simulink model "e4"  (R2016b)
settings: Solver=FixedStepDiscrete  StartTime=0.0  StopTime=inf  FixedStep=0.025  RelTol=1e-3  EnableMultiTasking=on
undefined symbols (not defined in the file or in its folder): codertarget, gcbh, sigbuilder_block
libraries: arduinolib x9, simulink x8, RASPlib x3, MinSegLibrary_M1V4 x3
settings Model: SimulationMode=external  ExtModeTrigDuration=2  Creator=Hamza  LastModifiedBy=Hamza
settings OptimizationCC: MaxStackSize=64
settings DebuggingCC: ParameterTunabilityLossMsg=error
settings HardwareCC: ProdBitPerPointer=32  ProdBitPerSizeT=32  ProdBitPerPtrDiffT=32  ProdLargestAtomicInteger=Long  ProdLargestAtomicFloat=Double  ProdWordSize=32  ProdHWDeviceType=ARM Compatible->ARM Cortex
settings RTWCC: SystemTargetFile=ert.tlc  HardwareBoard=Arduino Due  TLCOptions=-aInlineSetEventsForThisBaseRateFcn=TLC_FALSE -aSuppressMultiTaskScheduler=TLC_FALSE -aRateBasedStepFcn=1  TemplateMakefile=ert_default_tmf  Description=Embedded Coder  GenerateReport=on  Toolchain=Arduino ARM  BuildConfiguration=Faster Runs  IncludeHyperlinkInReport=on  LaunchReport=on  GenerateTraceInfo=on  GenerateTraceReport=on  GenerateTraceReportSl=on  GenerateTraceReportSf=on  GenerateTraceReportEml=on
settings CodeAppCC: ForceParamTrailComments=on  IgnoreCustomStorageClasses=off  OperatorAnnotations=on  SimulinkDataObjDesc=on  SFDataObjDesc=on  MATLABFcnDesc=on  InsertBlockDesc=on  MATLABSourceComments=on
settings ERTTargetCC: SupportContinuousTime=on  SupportVariableSizeSignals=on

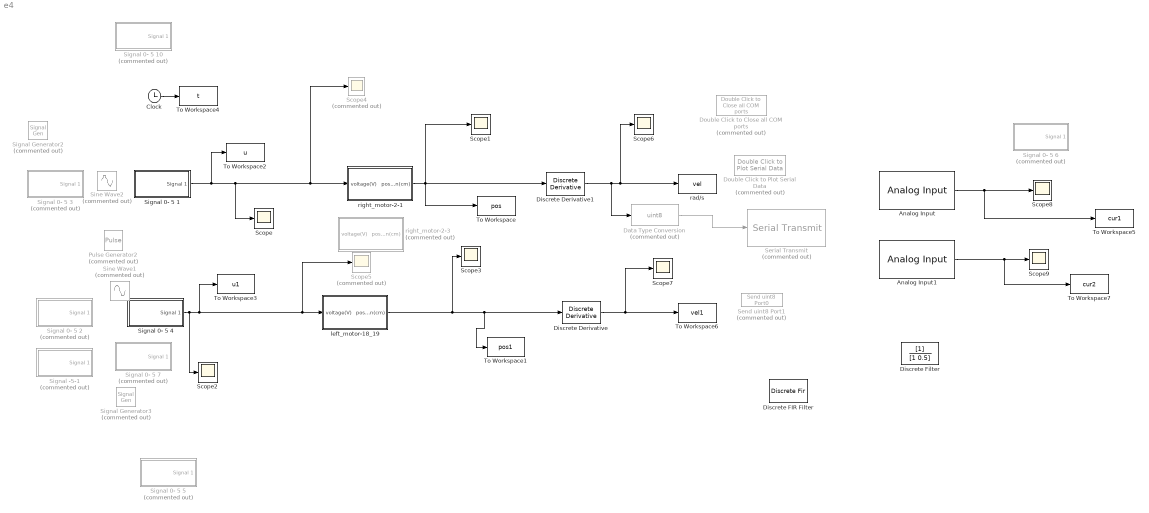
== system e4 ==
  Analog Input : arduinolib/Analog Input  pinNumber=0  sampleTime=0.025  blockPlatform=arduino
  Analog Input1 : arduinolib/Analog Input  pinNumber=1  sampleTime=0.025  blockPlatform=arduino
  Clock : Clock
  Data Type Conversion : DataTypeConversion  Commented=on  OutDataTypeStr=uint8
  Discrete Derivative : simulink/Discrete/Discrete Derivative  gainval=1.0  ICPrevScaledInput=0.0  OutMin=[]  OutMax=[]  OutDataType=fixdt(1, 16)  OutScaling=2^-10  DoSatur=off
  Discrete Derivative1 : simulink/Discrete/Discrete Derivative  gainval=1.0  ICPrevScaledInput=0.0  OutMin=[]  OutMax=[]  OutDataType=fixdt(1, 16)  OutScaling=2^-10  DoSatur=off
  Discrete FIR Filter : DiscreteFir
  Discrete Filter : DiscreteFilter
  Double Click to Close all COM ports : RASPlib/Double Click to Close all COM ports  Commented=on
  Double Click to Plot Serial Data : RASPlib/Double Click to Plot Serial Data  Commented=on  COMport=3  BaudRate=115200  NumSamples=10000  DataType=uint8
  Pulse Generator2 : DiscretePulseGenerator  Commented=on  PulseType=Time based  Amplitude=5  Period=20  PulseWidth=50  PhaseDelay=5
  Scope{,1..3,6..9} (8 alike) : Scope
  Scope4 : Scope  Commented=on
  Scope5 : Scope  Commented=on
  Send uint8 Port1 : RASPlib/Send uint8 Port0  Commented=on
  Serial Transmit : arduinolib/Serial Transmit  Commented=on  portNumber=0  blockPlatform=arduino
  Signal Generator2 : SignalGenerator  Commented=on  WaveForm=sawtooth  Amplitude=5  Frequency=0.05*pi  Units=rad/sec
  Signal Generator3 : SignalGenerator  Commented=on  WaveForm=sawtooth  Amplitude=-5  Frequency=0.05*pi  Units=rad/sec
  Signal -5-1 : Subsystem  Tag=STV Subsys  Commented=on  LoadFcn=sigbuilder_block('load');  StartFcn=sigbuilder_block('start');  StopFcn=sigbuilder_block('stop');  ClipboardFcn=sigbuilder_block('clipboard');  mask(Sigbuilder block){tuvar=[0:10]}
      mask help: Simulink:masks:SigbuilderBlock_MD
      mask init:
      | if ~strcmp(get_param(bdroot(gcbh),'SimulationStatus'),'stopped') tuvar = sigbuilder_block('maskInit'); end
      settings: CopyFcn=sigbuilder_block('copy');  DeleteFcn=sigbuilder_block('delete');  ModelCloseFcn=sigbuilder_block('modelClose');  PreSaveFcn=sigbuilder_block('preSave');  PauseFcn=sigbuilder_block('pause');  ContinueFcn=sigbuilder_block('continue');  NameChangeFcn=sigbuilder_block('namechange');  OpenFcn=sigbuilder_block('open',[6 30 1012.5 447.75 ]);  CloseFcn=sigbuilder_block('close');
      mask Display: plot(0, 0, 100, 100,[2, 2, 32, 32, 2], [68, 8, 8, 68, 68],[32, 2], [38, 38], [32, 19, 2],[53, 60, 44], [32, 17, 17, 2],[16, 16, 31, 31]);txt = getActiveGroup(gcbh);text(2, 100, txt,'verticalAlignment', 'top');
  Signal 0- 5 1 : Subsystem  Tag=STV Subsys  LoadFcn=sigbuilder_block('load');  StartFcn=sigbuilder_block('start');  StopFcn=sigbuilder_block('stop');  ClipboardFcn=sigbuilder_block('clipboard');  mask(Sigbuilder block){tuvar=[0:10]}
      mask help: Simulink:masks:SigbuilderBlock_MD
      mask init:
      | if ~strcmp(get_param(bdroot(gcbh),'SimulationStatus'),'stopped') tuvar = sigbuilder_block('maskInit'); end
      settings: CopyFcn=sigbuilder_block('copy');  DeleteFcn=sigbuilder_block('delete');  ModelCloseFcn=sigbuilder_block('modelClose');  PreSaveFcn=sigbuilder_block('preSave');  PauseFcn=sigbuilder_block('pause');  ContinueFcn=sigbuilder_block('continue');  NameChangeFcn=sigbuilder_block('namechange');  OpenFcn=sigbuilder_block('open',[6 30 1012.5 447.75 ]);  CloseFcn=sigbuilder_block('close');
      mask Display: plot(0, 0, 100, 100,[2, 2, 32, 32, 2], [68, 8, 8, 68, 68],[32, 2], [38, 38], [32, 19, 2],[53, 60, 44], [32, 17, 17, 2],[16, 16, 31, 31]);txt = getActiveGroup(gcbh);text(2, 100, txt,'verticalAlignment', 'top');
  Signal 0- 5 10 : Subsystem  Tag=STV Subsys  Commented=on  LoadFcn=sigbuilder_block('load');  StartFcn=sigbuilder_block('start');  StopFcn=sigbuilder_block('stop');  ClipboardFcn=sigbuilder_block('clipboard');  mask(Sigbuilder block){tuvar=[0:10]}
      mask help: Simulink:masks:SigbuilderBlock_MD
      mask init:
      | if ~strcmp(get_param(bdroot(gcbh),'SimulationStatus'),'stopped') tuvar = sigbuilder_block('maskInit'); end
      settings: CopyFcn=sigbuilder_block('copy');  DeleteFcn=sigbuilder_block('delete');  ModelCloseFcn=sigbuilder_block('modelClose');  PreSaveFcn=sigbuilder_block('preSave');  PauseFcn=sigbuilder_block('pause');  ContinueFcn=sigbuilder_block('continue');  NameChangeFcn=sigbuilder_block('namechange');  OpenFcn=sigbuilder_block('open',[6 30 1012.5 447.75 ]);  CloseFcn=sigbuilder_block('close');
      mask Display: plot(0, 0, 100, 100,[2, 2, 32, 32, 2], [68, 8, 8, 68, 68],[32, 2], [38, 38], [32, 19, 2],[53, 60, 44], [32, 17, 17, 2],[16, 16, 31, 31]);txt = getActiveGroup(gcbh);text(2, 100, txt,'verticalAlignment', 'top');
  Signal 0- 5 2 : Subsystem  Tag=STV Subsys  Commented=on  LoadFcn=sigbuilder_block('load');  StartFcn=sigbuilder_block('start');  StopFcn=sigbuilder_block('stop');  ClipboardFcn=sigbuilder_block('clipboard');  mask(Sigbuilder block){tuvar=[0:10]}
      mask help: Simulink:masks:SigbuilderBlock_MD
      mask init:
      | if ~strcmp(get_param(bdroot(gcbh),'SimulationStatus'),'stopped') tuvar = sigbuilder_block('maskInit'); end
      settings: CopyFcn=sigbuilder_block('copy');  DeleteFcn=sigbuilder_block('delete');  ModelCloseFcn=sigbuilder_block('modelClose');  PreSaveFcn=sigbuilder_block('preSave');  PauseFcn=sigbuilder_block('pause');  ContinueFcn=sigbuilder_block('continue');  NameChangeFcn=sigbuilder_block('namechange');  OpenFcn=sigbuilder_block('open',[6 30 1012.5 447.75 ]);  CloseFcn=sigbuilder_block('close');
      mask Display: plot(0, 0, 100, 100,[2, 2, 32, 32, 2], [68, 8, 8, 68, 68],[32, 2], [38, 38], [32, 19, 2],[53, 60, 44], [32, 17, 17, 2],[16, 16, 31, 31]);txt = getActiveGroup(gcbh);text(2, 100, txt,'verticalAlignment', 'top');
  Signal 0- 5 3 : Subsystem  Tag=STV Subsys  Commented=on  LoadFcn=sigbuilder_block('load');  StartFcn=sigbuilder_block('start');  StopFcn=sigbuilder_block('stop');  ClipboardFcn=sigbuilder_block('clipboard');  mask(Sigbuilder block){tuvar=[0:10]}
      mask help: Simulink:masks:SigbuilderBlock_MD
      mask init:
      | if ~strcmp(get_param(bdroot(gcbh),'SimulationStatus'),'stopped') tuvar = sigbuilder_block('maskInit'); end
      settings: CopyFcn=sigbuilder_block('copy');  DeleteFcn=sigbuilder_block('delete');  ModelCloseFcn=sigbuilder_block('modelClose');  PreSaveFcn=sigbuilder_block('preSave');  PauseFcn=sigbuilder_block('pause');  ContinueFcn=sigbuilder_block('continue');  NameChangeFcn=sigbuilder_block('namechange');  OpenFcn=sigbuilder_block('open',[6 30 1012.5 447.75 ]);  CloseFcn=sigbuilder_block('close');
      mask Display: plot(0, 0, 100, 100,[2, 2, 32, 32, 2], [68, 8, 8, 68, 68],[32, 2], [38, 38], [32, 19, 2],[53, 60, 44], [32, 17, 17, 2],[16, 16, 31, 31]);txt = getActiveGroup(gcbh);text(2, 100, txt,'verticalAlignment', 'top');
  Signal 0- 5 4 : Subsystem  Tag=STV Subsys  LoadFcn=sigbuilder_block('load');  StartFcn=sigbuilder_block('start');  StopFcn=sigbuilder_block('stop');  ClipboardFcn=sigbuilder_block('clipboard');  mask(Sigbuilder block){tuvar=[0:10]}
      mask help: Simulink:masks:SigbuilderBlock_MD
      mask init:
      | if ~strcmp(get_param(bdroot(gcbh),'SimulationStatus'),'stopped') tuvar = sigbuilder_block('maskInit'); end
      settings: CopyFcn=sigbuilder_block('copy');  DeleteFcn=sigbuilder_block('delete');  ModelCloseFcn=sigbuilder_block('modelClose');  PreSaveFcn=sigbuilder_block('preSave');  PauseFcn=sigbuilder_block('pause');  ContinueFcn=sigbuilder_block('continue');  NameChangeFcn=sigbuilder_block('namechange');  OpenFcn=sigbuilder_block('open',[6 30 1012.5 447.75 ]);  CloseFcn=sigbuilder_block('close');
      mask Display: plot(0, 0, 100, 100,[2, 2, 32, 32, 2], [68, 8, 8, 68, 68],[32, 2], [38, 38], [32, 19, 2],[53, 60, 44], [32, 17, 17, 2],[16, 16, 31, 31]);txt = getActiveGroup(gcbh);text(2, 100, txt,'verticalAlignment', 'top');
  Signal 0- 5 5 : Subsystem  Tag=STV Subsys  Commented=on  LoadFcn=sigbuilder_block('load');  StartFcn=sigbuilder_block('start');  StopFcn=sigbuilder_block('stop');  ClipboardFcn=sigbuilder_block('clipboard');  mask(Sigbuilder block){tuvar=[0:10]}
      mask help: Simulink:masks:SigbuilderBlock_MD
      mask init:
      | if ~strcmp(get_param(bdroot(gcbh),'SimulationStatus'),'stopped') tuvar = sigbuilder_block('maskInit'); end
      settings: CopyFcn=sigbuilder_block('copy');  DeleteFcn=sigbuilder_block('delete');  ModelCloseFcn=sigbuilder_block('modelClose');  PreSaveFcn=sigbuilder_block('preSave');  PauseFcn=sigbuilder_block('pause');  ContinueFcn=sigbuilder_block('continue');  NameChangeFcn=sigbuilder_block('namechange');  OpenFcn=sigbuilder_block('open',[6 30 1012.5 447.75 ]);  CloseFcn=sigbuilder_block('close');
      mask Display: plot(0, 0, 100, 100,[2, 2, 32, 32, 2], [68, 8, 8, 68, 68],[32, 2], [38, 38], [32, 19, 2],[53, 60, 44], [32, 17, 17, 2],[16, 16, 31, 31]);txt = getActiveGroup(gcbh);text(2, 100, txt,'verticalAlignment', 'top');
  Signal 0- 5 6 : Subsystem  Tag=STV Subsys  Commented=on  LoadFcn=sigbuilder_block('load');  StartFcn=sigbuilder_block('start');  StopFcn=sigbuilder_block('stop');  ClipboardFcn=sigbuilder_block('clipboard');  mask(Sigbuilder block){tuvar=[0:10]}
      mask help: Simulink:masks:SigbuilderBlock_MD
      mask init:
      | if ~strcmp(get_param(bdroot(gcbh),'SimulationStatus'),'stopped') tuvar = sigbuilder_block('maskInit'); end
      settings: CopyFcn=sigbuilder_block('copy');  DeleteFcn=sigbuilder_block('delete');  ModelCloseFcn=sigbuilder_block('modelClose');  PreSaveFcn=sigbuilder_block('preSave');  PauseFcn=sigbuilder_block('pause');  ContinueFcn=sigbuilder_block('continue');  NameChangeFcn=sigbuilder_block('namechange');  OpenFcn=sigbuilder_block('open',[6 30 1012.5 447.75 ]);  CloseFcn=sigbuilder_block('close');
      mask Display: plot(0, 0, 100, 100,[2, 2, 32, 32, 2], [68, 8, 8, 68, 68],[32, 2], [38, 38], [32, 19, 2],[53, 60, 44], [32, 17, 17, 2],[16, 16, 31, 31]);txt = getActiveGroup(gcbh);text(2, 100, txt,'verticalAlignment', 'top');
  Signal 0- 5 7 : Subsystem  Tag=STV Subsys  Commented=on  LoadFcn=sigbuilder_block('load');  StartFcn=sigbuilder_block('start');  StopFcn=sigbuilder_block('stop');  ClipboardFcn=sigbuilder_block('clipboard');  mask(Sigbuilder block){tuvar=[0:10]}
      mask help: Simulink:masks:SigbuilderBlock_MD
      mask init:
      | if ~strcmp(get_param(bdroot(gcbh),'SimulationStatus'),'stopped') tuvar = sigbuilder_block('maskInit'); end
      settings: CopyFcn=sigbuilder_block('copy');  DeleteFcn=sigbuilder_block('delete');  ModelCloseFcn=sigbuilder_block('modelClose');  PreSaveFcn=sigbuilder_block('preSave');  PauseFcn=sigbuilder_block('pause');  ContinueFcn=sigbuilder_block('continue');  NameChangeFcn=sigbuilder_block('namechange');  OpenFcn=sigbuilder_block('open',[6 30 1012.5 447.75 ]);  CloseFcn=sigbuilder_block('close');
      mask Display: plot(0, 0, 100, 100,[2, 2, 32, 32, 2], [68, 8, 8, 68, 68],[32, 2], [38, 38], [32, 19, 2],[53, 60, 44], [32, 17, 17, 2],[16, 16, 31, 31]);txt = getActiveGroup(gcbh);text(2, 100, txt,'verticalAlignment', 'top');
  Sine Wave1 : Sin  Commented=on  Amplitude=5  Frequency=0.4*3.14  Phase=pi
  Sine Wave2 : Sin  Commented=on  Amplitude=5  Frequency=0.4*pi
  To Workspace : ToWorkspace  VariableName=pos  SampleTime=-1
      settings: Save2DSignal=2-D array (concatenate along first dimension)
  To Workspace1 : ToWorkspace  VariableName=pos1  SampleTime=-1
      settings: Save2DSignal=2-D array (concatenate along first dimension)
  To Workspace2 : ToWorkspace  VariableName=u  SampleTime=-1
      settings: Save2DSignal=2-D array (concatenate along first dimension)
  To Workspace3 : ToWorkspace  VariableName=u1  SampleTime=-1
      settings: Save2DSignal=2-D array (concatenate along first dimension)
  To Workspace4 : ToWorkspace  VariableName=t  SampleTime=-1
      settings: Save2DSignal=2-D array (concatenate along first dimension)
  To Workspace5 : ToWorkspace  VariableName=cur1  SampleTime=-1
      settings: Save2DSignal=2-D array (concatenate along first dimension)
  To Workspace6 : ToWorkspace  VariableName=vel1  SampleTime=-1
      settings: Save2DSignal=2-D array (concatenate along first dimension)
  To Workspace7 : ToWorkspace  VariableName=cur2  SampleTime=-1
      settings: Save2DSignal=2-D array (concatenate along first dimension)
  "left_motor-18_19 " : Subsystem
  rad/s : ToWorkspace  VariableName=vel  SampleTime=-1
      settings: Save2DSignal=2-D array (concatenate along first dimension)
  right_motor-2-1 : Subsystem
  right_motor-2-3 : Subsystem  Commented=on
  wires:
  right_motor-2-1/1(position(cm)) -> To Workspace/1, Scope1/1, Discrete Derivative1/1
  "left_motor-18_19 "/1(position(cm)) -> Discrete Derivative/1, To Workspace1/1, Scope3/1
  Signal 0- 5 4/1(Signal 1) -> Scope2/1, Scope5/1, "left_motor-18_19 "/1(voltage(V)), To Workspace3/1
  Clock/1 -> To Workspace4/1
  Discrete Derivative/1 -> Scope7/1, To Workspace6/1
  Discrete Derivative1/1 -> Data Type Conversion/1, Scope6/1, rad/s/1
  Data Type Conversion/1 -> Serial Transmit/1
  Signal 0- 5 1/1(Signal 1) -> To Workspace2/1, Scope/1, right_motor-2-1/1(voltage(V)), Scope4/1
  Analog Input/1 -> To Workspace5/1, Scope8/1
  Analog Input1/1 -> To Workspace7/1, Scope9/1

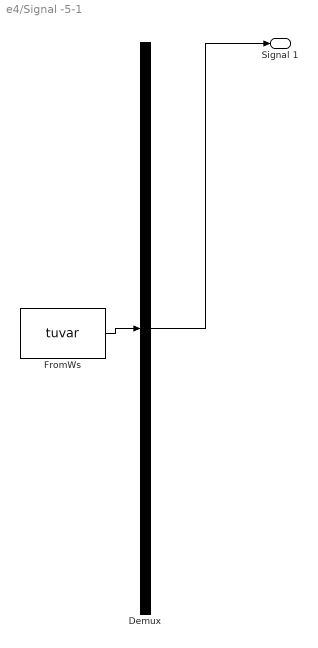
== system e4/Signal -5-1 ==
  Demux : Demux  Tag=STV Demux  Outputs=1
  FromWs : FromWorkspace  Tag=STV FromWs  VariableName=tuvar  SampleTime=0
      SigBuilderData=|
      | common.afterFinalStr = 'Extrapolate'
      | common.sampleTime = 0
      | dataSet.timeRange = [0 60]
      | dataSet.name = 'Group 1'
      | sbobj.Groups.Name = 'Group 1'
      | sbobj.Groups.Signals.Name = 'Signal 1'
      | sbobj.Groups.Signals.XData = [0 5 5 9.99 9.99 15 15 20.005 20.005 25 25 30 30 34.95 34.95 40 40 45 45 50 50 55 55 60]
      | sbobj.Groups.Signals.YData = [0 0 -5 -5 -4.5 -4.5 -4 -4 -3.49 -3.49 -3.01 -3.01 -2.49 -2.49 -2 -2 -1.5 -1.5 -1.01 -1.01 -0.5 -0.5 0 0]
      | sbobj.Groups.TimeRange = [0 60]
  Signal 1 : Outport  Tag=STV Outport
  wires:
  FromWs/1 -> Demux/1
  Demux/1 -> Signal 1/1

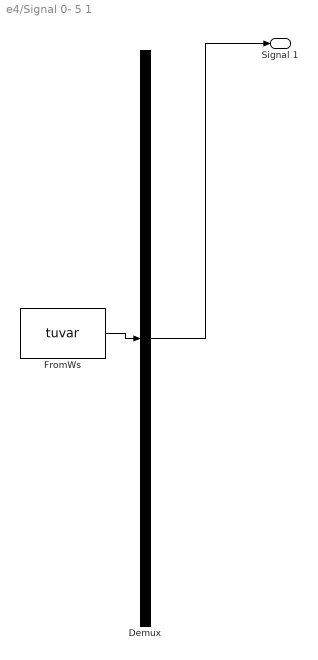
== system e4/Signal 0- 5 1 ==
  Demux : Demux  Tag=STV Demux  Outputs=1
  FromWs : FromWorkspace  Tag=STV FromWs  VariableName=tuvar  SampleTime=0
      SigBuilderData=|
      | common.afterFinalStr = 'Extrapolate'
      | common.sampleTime = 0
      | dataSet.timeRange = [0 150]
      | dataSet.name = 'Group 1'
      | sbobj.Groups.Name = 'Group 1'
      | sbobj.Groups.Signals.Name = 'Signal 1'
      | sbobj.Groups.Signals.XData = [0 5 10 15 20 25 30 35 40 45 47.5 50 52.5 55 57.5 60 62.5 70 75 80 85 90 95 100 105 150]
      | sbobj.Groups.Signals.YData = [0 0 5 5 0 0 -5 -5 0 0 5 5 0 0 -5 -5 0 0 -5 -5 0 0 5 5 0 0]
      | sbobj.Groups.TimeRange = [0 150]
  Signal 1 : Outport  Tag=STV Outport
  wires:
  FromWs/1 -> Demux/1
  Demux/1 -> Signal 1/1

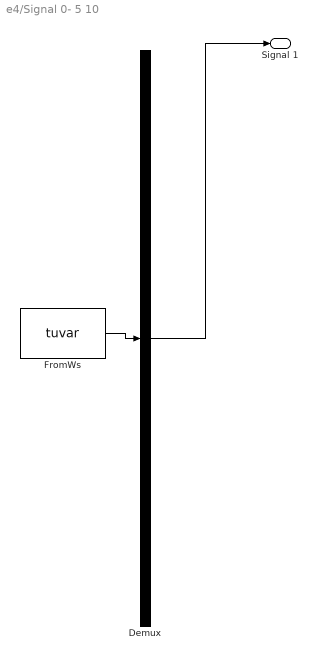
== system e4/Signal 0- 5 10 ==
  Demux : Demux  Tag=STV Demux  Outputs=1
  FromWs : FromWorkspace  Tag=STV FromWs  VariableName=tuvar  SampleTime=0
      SigBuilderData=|
      | common.afterFinalStr = 'Extrapolate'
      | common.sampleTime = 0
      | dataSet.timeRange = [0 1700]
      | dataSet.name = 'Group 1'
      | sbobj.Groups.Name = 'Group 1'
      | sbobj.Groups.Signals.Name = 'Signal 1'
      | sbobj.Groups.Signals.XData = [0 10 10 20 20 30 30 40 40 50 50 60 60 70 70 80 80 90 90 100 100 110 110 120 120 130 130 140 140 150 150 160 160 170 170 180 180 190 190 200 200 210 210 220 220 230 230 240 240 250 250 260 260 270 270 280 280 290 290 300 300 310 310 320 320 330 330 340 340 350 350 360 360 370 370 380 380 390 390 400 400 410 410 420 420 430 430 440 440 450 450 460 460 470 470 480 480 490 490 500 500 510 510 520 520 530 540 540 550 550 560 560 570 570 580 580 590 590 600 600 610 610 620 620 630 630 640 640 650 650 660 660 670 670 680 680 690 690 700 700 710 710 720 720 730 730 740 740 750 750 760 760 770 770 780 780 790 790 800 800 810 810 820 820 830 830 840 840 850 850 860 860 870 870 880 880 890 890 900 900 910 910 920 920 930 930 940 940 950 950 960 960 970 970 980 980 990 990 1000 1000 1010 1010 1020 1020 1030 1030 1040 1040 1050 1050 1060 1060 1070 1070 1080 1080 1090 1090 1100 1100 1110 1110 1120 1120 1130 1130 1140 1140 1150 1150 1160 1160 1170 1170 1180 1180 1190 1190 1200 1200 1210 1210 1220 1220 1230 1230 1240 1240 1250 1250 1260 1260 1270 1270 1280 1280 1290 1290 1300 1300 1310 1310 1320 1320 1330 1330 1340 1340 1350 1350 1360 1360 1370 1370 1380 1380 1390 1390 1400 1400 1410 1410 1420 1420 1430 1430 1440 1440 1450 1450 1460 1460 1470 1470 1480 1480 1490 1490 1500 1500 1510 1510 1520 1520 1530 1530 1540 1540 1550 1550 1560 1560 1570 1570 1580 1580 1590 1590 1600 1600 1610 1610 1620 1620 1630 1630 1700]
      | sbobj.Groups.Signals.YData = [0 0 -5 -5 0 0 -4.8 -4.8 0 0 -4.6 -4.6 0 0 -4.4 -4.4 0 0 -4.2 -4.2 0 0 -4 -4 0 0 -3.8 -3.8 0 0 -3.6 -3.6 0 0 -3.4 -3.4 0 0 -3.2 -3.2 0 0 -3 -3 0 0 -2.9 -2.9 0 0 -2.8 -2.8 0 0 -2.7 -2.7 0 0 -2.6 -2.6 0 0 -2.5 -2.5 0 0 -2.4 -2.4 0 0 -2.3 -2.3 0 0 -2.2 -2.2 0 0 -2.1 -2.1 0 0 -2 -2 0 0 -1.9 -1.9 0 0 -1.8 -1.8 0 0 -1.7 -1.7 0 0 -1.6 -1.6 0 0 -1.5 -1.5 0 0 0 -1.4 -1.4 0 0 -1.3 -1.3 0 0 -1.2 -1.2 0 0 -1.1 -1.1 0 0 -1 -1 0 0 -0.9 -0.9 0 0 -0.8 -0.8 0 0 -0.7 -0.7 0 0 -0.6 -0.6 0 0 -0.5 -0.5 0 0 -0.4 -0.4 0 0 -0.3 -0.3 0 0 -0.2 -0.2 0 0 -0.1 -0.1 0 0 5 5 0 0 0.1 0.1 0 0 0.2 0.2 0 0 0.3 0.3 0 0 0.4 0.4 0 0 0.5 0.5 0 0 0.6 0.6 0 0 0.7 0.7 0 0 0.8 0.8 0 0 0.9 0.9 0 0 1 1 0 0 1.1 1.1 0 0 1.2 1.2 0 0 1.3 1.3 0 0 1.4 1.4 0 0 1.5 1.5 0 0 1.6 1.6 0 0 1.7 1.7 0 0 1.8 1.8 0 0 1.9 1.9 0 0 2 2 0 0 2.1 2.1 0 0 2.2 2.2 0 0 2.3 2.3 0 0 2.4 2.4 0 0 2.5 2.5 0 0 2.6 2.6 0 0 2.7 2.7 0 0 2.8 2.8 0 0 2.9 2.9 0 0 3 3 0 0 3.2 3.2 0 0 3.4 3.4 0 0 3.6 3.6 0 0 3.8 3.8 0 0 4 4 0 0 4.2 4.2 0 0 4.4 4.4 0 0 4.6 4.6 0 0 4.8 4.8 0 0 5 5 0 0]
      | sbobj.Groups.TimeRange = [0 1700]
  Signal 1 : Outport  Tag=STV Outport
  wires:
  Demux/1 -> Signal 1/1
  FromWs/1 -> Demux/1

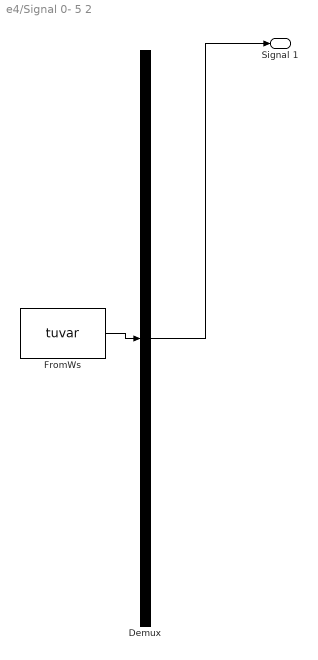
== system e4/Signal 0- 5 2 ==
  Demux : Demux  Tag=STV Demux  Outputs=1
  FromWs : FromWorkspace  Tag=STV FromWs  VariableName=tuvar  SampleTime=0
      SigBuilderData=|
      | common.afterFinalStr = 'Extrapolate'
      | common.sampleTime = 0
      | dataSet.timeRange = [0 600]
      | dataSet.name = 'Group 1'
      | sbobj.Groups.Name = 'Group 1'
      | sbobj.Groups.Signals.Name = 'Signal 1'
      | sbobj.Groups.Signals.XData = [0 10 10 20 20 29.99 29.99 40 40 50 50 60 60 70 70 80 80 90 90 100 100 109.95 109.95 120.05 120.05 130.05 130.05 139.98 139.98 150 150 159.95 159.95 170 170 180 180 190 190 200 200 210 210 220 220 230 230 240 240 249.98 249.98 260 260 270 270 280 280 289.95 289.95 300 300 310 310 320 320 330 330 340 340 350 350 360.05 360.05 370 370 380 380 390 390 400 400 410 410 420 420 430.05 430.05 440.05 440.05 449.95 449.95 460 460 470 470 480 480 489.95 489.95 500 500 520.1 529.9 540.1 550 560.1 569.95 580 580 600]
      | sbobj.Groups.Signals.YData = [0 0 0.1 0.1 0.2 0.2 0.3 0.3 0.4 0.4 0.5 0.5 0.602 0.602 0.7 0.7 0.8 0.8 0.902 0.902 1 1 1.102 1.102 1.2 1.2 1.3 1.3 1.4 1.4 1.5 1.5 1.6 1.6 1.7 1.7 1.802 1.802 1.9 1.9 2 2 2.1 2.1 2.202 2.202 2.3 2.3 2.404 2.404 2.5 2.5 2.598 2.598 2.7 2.7 2.8 2.8 2.9 2.9 3 3 3.102 3.102 3.2 3.2 3.3 3.3 3.4 3.4 3.5 3.5 3.6 3.6 3.7 3.7 3.798 3.798 3.9 3.9 3.998 3.998 4.102 4.102 4.198 4.198 4.3 4.3 4.402 4.402 4.502 4.502 4.6 4.6 4.7 4.7 4.798 4.798 4.9 4.9 5 5 5 5 5 5 5 5 0 0]
      | sbobj.Groups.TimeRange = [0 600]
  Signal 1 : Outport  Tag=STV Outport
  wires:
  FromWs/1 -> Demux/1
  Demux/1 -> Signal 1/1

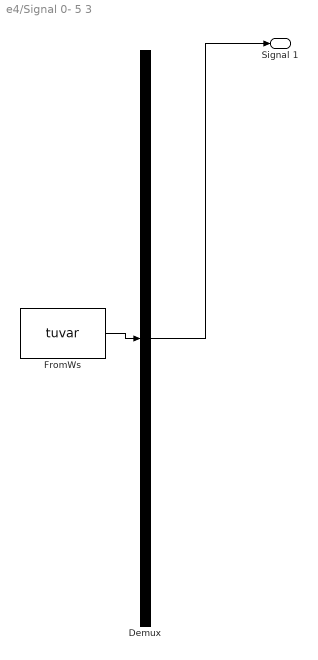
== system e4/Signal 0- 5 3 ==
  Demux : Demux  Tag=STV Demux  Outputs=1
  FromWs : FromWorkspace  Tag=STV FromWs  VariableName=tuvar  SampleTime=0
      SigBuilderData=|
      | common.afterFinalStr = 'Extrapolate'
      | common.sampleTime = 0
      | dataSet.timeRange = [0 120]
      | dataSet.name = 'Group 1'
      | sbobj.Groups.Name = 'Group 1'
      | sbobj.Groups.Signals.Name = 'Signal 1'
      | sbobj.Groups.Signals.XData = [0 10 10 20 20 29.95 29.95 40 40 50.05 50.05 60 60 70.05 70.05 79.95 79.95 90 90 99.95 99.95 118.85 118.85 120]
      | sbobj.Groups.Signals.YData = [0 0 0.49 0.49 1.005 1.005 1.5 1.5 1.99 1.98 2.49 2.488 3.01 3.007525 3.5 3.49322259136 4 3.98 4.5 4.5 4.98 4.98 0 0]
      | sbobj.Groups.TimeRange = [0 120]
  Signal 1 : Outport  Tag=STV Outport
  wires:
  Demux/1 -> Signal 1/1
  FromWs/1 -> Demux/1

== system e4/Signal 0- 5 4 ==
  Demux : Demux  Tag=STV Demux  Outputs=1
  FromWs : FromWorkspace  Tag=STV FromWs  VariableName=tuvar  SampleTime=0
      SigBuilderData=|
      | common.afterFinalStr = 'Extrapolate'
      | common.sampleTime = 0
      | dataSet.timeRange = [0 150]
      | dataSet.name = 'Group 1'
      | sbobj.Groups.Name = 'Group 1'
      | sbobj.Groups.Signals.Name = 'Signal 1'
      | sbobj.Groups.Signals.XData = [0 5 10 15 20 25 30 35 40 45 47.5 50 52.5 55 57.5 60 62.5 70 75 80 85 90 95 100 105 150]
      | sbobj.Groups.Signals.YData = [0 0 -5 -5 0 0 5 5 0 0 5 5 0 0 -5 -5 0 0 5 5 0 0 -5 -5 0 0]
      | sbobj.Groups.TimeRange = [0 150]
  Signal 1 : Outport  Tag=STV Outport
  wires:
  Demux/1 -> Signal 1/1
  FromWs/1 -> Demux/1

== system e4/Signal 0- 5 5 ==
  Demux : Demux  Tag=STV Demux  Outputs=1
  FromWs : FromWorkspace  Tag=STV FromWs  VariableName=tuvar  SampleTime=0
      SigBuilderData=|
      | common.afterFinalStr = 'Extrapolate'
      | common.sampleTime = 0
      | dataSet.timeRange = [0 1000]
      | dataSet.name = 'Group 1'
      | sbobj.Groups.Name = 'Group 1'
      | sbobj.Groups.Signals.Name = 'Signal 1'
      | sbobj.Groups.Signals.XData = [0 10 10 20 20 29.99 29.99 40 40 50 50 60 60 70 70 80 80 90 90 100 100 109.95 109.95 120.05 120.05 130.05 130.05 139.98 139.98 150 150 159.95 159.95 170 170 180 180 190 190 200 200 210 210 220 220 230 230 240 240 249.98 249.98 260 260 270 270 280 280 289.95 289.95 300 300 310 310 320 320 330 330 340 340 350 350 360.05 360.05 370 370 380 380 390 390 400 400 410 410 420 420 430.05 430.05 440.05 440.05 449.95 449.95 460 460 470 470 480 480 489.95 489.95 500 500 520.1 520.1 529.9 529.9 540.02 540.02 550 550 560.02 560.02 569.95 569.95 580 580 589.9 589.9 600 600 610 610 620 620 630 630 640 640 650 650 660 660 670 670 680 680 689.9 689.9 700 700 709.95 709.95 720 720 730 730 740 740 750 750 759.95 759.95 770 770 779.95 779.95 789.95 789.95 800 800 810 810 820 820 830 830 840 840 850 850 860 860 870 870 880 880 890 890 900.05 900.05 910.1 910.1 920 920 929.95 929.95 940 940 950.05 950.05 959.95 959.95 969.95 969.95 980 980 989.98 989.98 1000]
      | sbobj.Groups.Signals.YData = [0 0 0.1 0.1 0 0 0.3 0.3 0 0 0.5 0.5 0 0 0.7 0.7 -0.02 -0.02 0.902 0.902 -0.002 -0.002 1.102 1.102 0 0 1.3 1.3 0 0 1.5 1.5 0 0 1.7 1.7 -0.02 -0.02 1.9 1.9 0 0 2.1 2.1 0 0 2.3 2.3 0 0 2.5 2.5 -0.002 -0.002 2.7 2.7 0 0 2.9 2.9 -0.02 -0.02 3.102 3.102 -0.02 -0.02 3.3 3.3 0 0 3.5 3.5 -0.02 -0.02 3.7 3.7 0 0 3.9 3.9 -0.02 -0.02 4.102 4.102 -0.02 -0.02 4.3 4.3 -0.02 -0.02 4.502 4.502 0 0 4.7 4.7 0 0 5 5 0 0 -0.2 -0.2 0 0 -0.4 -0.4 0 0 -0.601 -0.601 0 0 -0.78 -0.78 0 0 -1 -1 0 0 -1.2 -1.2 0 0 -1.398 -1.398 0 0 -1.6 -1.6 0 0 -1.795 -1.795 0 0 -2 -2 0 0 -2.195 -2.195 0 0 -2.405 -2.405 0 0 -2.6 -2.6 0 0 -2.798 -2.798 0 0 -3 -3 0 0 -3.3 -3.3 0 0 -3.6 -3.6 0 0 -3.8 -3.8 0 0 -3.998 -3.998 0 0 -4.2 -4.2 0 0 -4.4 -4.4 0 0 -4.6 -4.6 0 0 -4.804 -4.804 0 0 -5 -5 0 0]
      | sbobj.Groups.TimeRange = [0 1000]
  Signal 1 : Outport  Tag=STV Outport
  wires:
  FromWs/1 -> Demux/1
  Demux/1 -> Signal 1/1

== system e4/Signal 0- 5 6 ==
  Demux : Demux  Tag=STV Demux  Outputs=1
  FromWs : FromWorkspace  Tag=STV FromWs  VariableName=tuvar  SampleTime=0
      SigBuilderData=|
      | common.afterFinalStr = 'Extrapolate'
      | common.sampleTime = 0
      | dataSet.timeRange = [0 150]
      | dataSet.name = 'Group 1'
      | sbobj.Groups.Name = 'Group 1'
      | sbobj.Groups.Signals.Name = 'Signal 1'
      | sbobj.Groups.Signals.XData = [0 25 30 35 40 65 70 75 80 150]
      | sbobj.Groups.Signals.YData = [0 0 -5 -5 0 0 5 5 0 0]
      | sbobj.Groups.TimeRange = [0 150]
  Signal 1 : Outport  Tag=STV Outport
  wires:
  Demux/1 -> Signal 1/1
  FromWs/1 -> Demux/1

== system e4/Signal 0- 5 7 ==
  Demux : Demux  Tag=STV Demux  Outputs=1
  FromWs : FromWorkspace  Tag=STV FromWs  VariableName=tuvar  SampleTime=0
      SigBuilderData=|
      | common.afterFinalStr = 'Extrapolate'
      | common.sampleTime = 0
      | dataSet.timeRange = [0 120]
      | dataSet.name = 'Group 1'
      | sbobj.Groups.Name = 'Group 1'
      | sbobj.Groups.Signals.Name = 'Signal 1'
      | sbobj.Groups.Signals.XData = [0 10 20 29.95 40 50.05 60 70 79.95 90 99.95 118.85 118.85 120]
      | sbobj.Groups.Signals.YData = [0 0 -5 -5 0 0 5 5 -0.05 -0.05 -0.05 -0.05 0 0]
      | sbobj.Groups.TimeRange = [0 120]
  Signal 1 : Outport  Tag=STV Outport
  wires:
  Demux/1 -> Signal 1/1
  FromWs/1 -> Demux/1

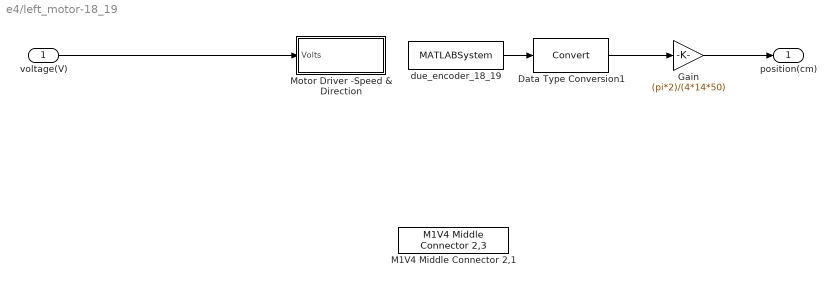
== system e4/left_motor-18_19  ==
  voltage(V) : Inport
  Data Type Conversion1 : DataTypeConversion
  Gain : Gain  Gain=(pi*2)/(4*14*50)
  M1V4 Middle Connector 2,1 : MinSegLibrary_M1V4/M1V4 Middle Connector 2,3  Encoder=1  PinA=18  PinB=19  PWMFSelect=1  PWMTimer=-1  SampleTime=-1
  Motor Driver -Speed & Direction : Subsystem  AncestorBlock=RASPlib/Motor Driver -Speed & Direction  mask(Motor Driver){Vsupply=5, PWMPin=5, DigitalPin=4}
      mask prompts: Vsupply "Driver Voltage"; PWMPin "PWM Pin"; DigitalPin "Digital Pin"
      mask help:
      | Use a single PWM and a single Digtial out to control the magnitude and direction of a motor
      |
      | Specify driver supply voltage (3.25 for USB with SN754410)
      mask Display:
      | port_label('input',1,'Volts')
      | text(15,5,['Vsupply=' num2str(Vsupply)])
  "due_encoder_18_19 " : MATLABSystem  System=Encoder_arduino_Due_18_19  Encoder=1  PinA=18  PinB=19  PWMFSelect=1  PWMTimer=-1  SampleTime=-1
      mask Type: Encoder_arduino_Due_18_19
      mask Display:
      | disp('soEncoder');
      | port_label('output',1,'y');
  position(cm) : Outport
  wires:
  voltage(V)/1 -> Motor Driver -Speed & Direction/1(Volts)
  "due_encoder_18_19 "/1 -> Data Type Conversion1/1
  Data Type Conversion1/1 -> Gain/1
  Gain/1 -> position(cm)/1

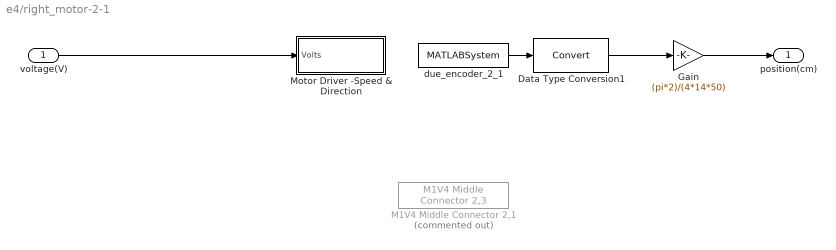
== system e4/right_motor-2-1 ==
  voltage(V) : Inport
  Data Type Conversion1 : DataTypeConversion
  Gain : Gain  Gain=(pi*2)/(4*14*50)
  M1V4 Middle Connector 2,1 : MinSegLibrary_M1V4/M1V4 Middle Connector 2,3  Commented=on  Encoder=0  PinA=2  PinB=3  PWMFSelect=1  PWMTimer=-1  SampleTime=-1
  Motor Driver -Speed & Direction : Subsystem  AncestorBlock=RASPlib/Motor Driver -Speed & Direction  mask(Motor Driver){Vsupply=5, PWMPin=5, DigitalPin=4}
      mask prompts: Vsupply "Driver Voltage"; PWMPin "PWM Pin"; DigitalPin "Digital Pin"
      mask help:
      | Use a single PWM and a single Digtial out to control the magnitude and direction of a motor
      |
      | Specify driver supply voltage (3.25 for USB with SN754410)
      mask Display:
      | port_label('input',1,'Volts')
      | text(15,5,['Vsupply=' num2str(Vsupply)])
  due_encoder_2_1 : MATLABSystem  System=Encoder_arduino_Due_2_3  Encoder=0  PinA=2  PinB=3  PWMFSelect=1  PWMTimer=-1  SampleTime=-1
      mask Type: Encoder_arduino_Due_2_3
      mask Display:
      | disp('soEncoder');
      | port_label('output',1,'y');
  position(cm) : Outport
  wires:
  Gain/1 -> position(cm)/1
  Data Type Conversion1/1 -> Gain/1
  due_encoder_2_1/1 -> Data Type Conversion1/1
  voltage(V)/1 -> Motor Driver -Speed & Direction/1(Volts)

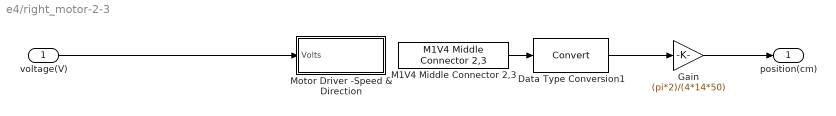
== system e4/right_motor-2-3 ==
  voltage(V) : Inport
  Data Type Conversion1 : DataTypeConversion
  Gain : Gain  Gain=(pi*2)/(4*14*50)
  M1V4 Middle Connector 2,3 : MinSegLibrary_M1V4/M1V4 Middle Connector 2,3  Encoder=0  PinA=2  PinB=3  PWMFSelect=1  PWMTimer=-1  SampleTime=-1
  Motor Driver -Speed & Direction : Subsystem  AncestorBlock=RASPlib/Motor Driver -Speed & Direction  mask(Motor Driver){Vsupply=5, PWMPin=5, DigitalPin=4}
      mask prompts: Vsupply "Driver Voltage"; PWMPin "PWM Pin"; DigitalPin "Digital Pin"
      mask help:
      | Use a single PWM and a single Digtial out to control the magnitude and direction of a motor
      |
      | Specify driver supply voltage (3.25 for USB with SN754410)
      mask Display:
      | port_label('input',1,'Volts')
      | text(15,5,['Vsupply=' num2str(Vsupply)])
  position(cm) : Outport
  wires:
  Gain/1 -> position(cm)/1
  Data Type Conversion1/1 -> Gain/1
  M1V4 Middle Connector 2,3/1 -> Data Type Conversion1/1
  voltage(V)/1 -> Motor Driver -Speed & Direction/1(Volts)

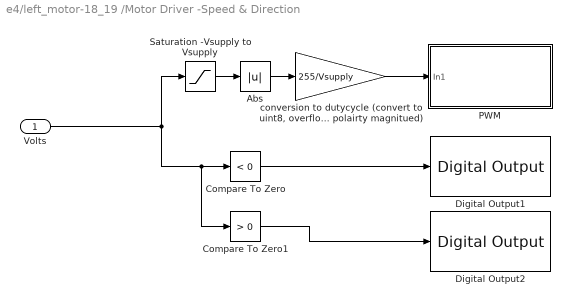
== system e4/left_motor-18_19 /Motor Driver -Speed & Direction ==
  Volts : Inport
  Abs : Abs
  Compare To Zero : simulink/Logic and Bit Operations/Compare To Zero  relop=<  OutDataTypeStr=boolean
  Compare To Zero1 : simulink/Logic and Bit Operations/Compare To Zero  relop=>  OutDataTypeStr=boolean
  Digital Output1 : arduinolib/Digital Output  pinNumber=8  blockPlatform=arduino
  Digital Output2 : arduinolib/Digital Output  pinNumber=7  blockPlatform=arduino
  PWM : Subsystem  AncestorBlock=arduinolib/PWM  InitFcn=codertarget.arduinobase.blocks.arduinoBlockInitFcnCallback(gcbh);  mask(Arduino PWM){pinNumber=9, blockPlatform=arduino}
      mask prompts: pinNumber "Pin number:"; blockPlatform "Block platform:"
      mask help:
      | Generate square waveform on the specified analog output pin. The block input controls the duty cycle of the square waveform. An input value of 0 produces a 0 percent duty cycle, and an input value of 255 produces a 100 percent duty cycle. The frequency of the waveform is constant at approximately 490 Hz.
      |
      | Enter the number of the analog output pin. Do not assign the same pin number to multiple blocks within a model.
      mask init:
      | codertarget.arduinobase.blocks.registerPWMBlock(gcbh);
      | codertarget.arduinobase.blocks.arduinoAnalogOutputCallback('MaskInitialization');
      mask Help: eval('codertarget.internal.helpView(''arduinoert'', ''arduinolibarduinopwm'')')
      mask DialogControl Control2 Prompt: View pin map
      mask DialogControl Control2 Callback:
      | file = [codertarget.arduinobase.internal.getBaseSpPkgRootDir filesep 'blocks' filesep 'mex' filesep 'arduinoPinMapping.html'];
      | web(file)
      mask Display:
      | pic=imread('analogoutpwm.png');image(pic,[0.32 0.25 0.35 0.55]);text(0.5, 0.15, 'Pin 9', 'horizontalAlignment', 'center');
      | color('blue');
      | text(0.55, 0.87, 'ARDUINO', 'horizontalAlignment', 'left');
      | color('black');
  Saturation -Vsupply to Vsupply : Saturate  UpperLimit=5  LowerLimit=-5  OutDataTypeStr=single
  "conversion to dutycycle (convert to uint8, overflow will provide reverse polairty magnitued)" : Gain  Gain=255/Vsupply  OutDataTypeStr=uint8
  wires:
  Volts/1 -> Compare To Zero1/1, Compare To Zero/1, Saturation -Vsupply to Vsupply/1
  Saturation -Vsupply to Vsupply/1 -> Abs/1
  "conversion to dutycycle (convert to uint8, overflow will provide reverse polairty magnitued)"/1 -> PWM/1(In1)
  Compare To Zero/1 -> Digital Output1/1
  Compare To Zero1/1 -> Digital Output2/1
  Abs/1 -> "conversion to dutycycle (convert to uint8, overflow will provide reverse polairty magnitued)"/1

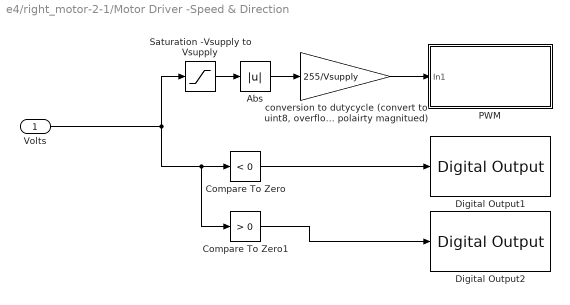
== system e4/right_motor-2-1/Motor Driver -Speed & Direction ==
  Volts : Inport
  Abs : Abs
  Compare To Zero : simulink/Logic and Bit Operations/Compare To Zero  relop=<  OutDataTypeStr=boolean
  Compare To Zero1 : simulink/Logic and Bit Operations/Compare To Zero  relop=>  OutDataTypeStr=boolean
  Digital Output1 : arduinolib/Digital Output  pinNumber=6  blockPlatform=arduino
  Digital Output2 : arduinolib/Digital Output  pinNumber=5  blockPlatform=arduino
  PWM : Subsystem  AncestorBlock=arduinolib/PWM  InitFcn=codertarget.arduinobase.blocks.arduinoBlockInitFcnCallback(gcbh);  mask(Arduino PWM){pinNumber=4, blockPlatform=arduino}
      mask prompts: pinNumber "Pin number:"; blockPlatform "Block platform:"
      mask help:
      | Generate square waveform on the specified analog output pin. The block input controls the duty cycle of the square waveform. An input value of 0 produces a 0 percent duty cycle, and an input value of 255 produces a 100 percent duty cycle. The frequency of the waveform is constant at approximately 490 Hz.
      |
      | Enter the number of the analog output pin. Do not assign the same pin number to multiple blocks within a model.
      mask init:
      | codertarget.arduinobase.blocks.registerPWMBlock(gcbh);
      | codertarget.arduinobase.blocks.arduinoAnalogOutputCallback('MaskInitialization');
      mask Help: eval('codertarget.internal.helpView(''arduinoert'', ''arduinolibarduinopwm'')')
      mask DialogControl Control2 Prompt: View pin map
      mask DialogControl Control2 Callback:
      | file = [codertarget.arduinobase.internal.getBaseSpPkgRootDir filesep 'blocks' filesep 'mex' filesep 'arduinoPinMapping.html'];
      | web(file)
      mask Display:
      | pic=imread('analogoutpwm.png');image(pic,[0.32 0.25 0.35 0.55]);text(0.5, 0.15, 'Pin 4', 'horizontalAlignment', 'center');
      | color('blue');
      | text(0.55, 0.87, 'ARDUINO', 'horizontalAlignment', 'left');
      | color('black');
  Saturation -Vsupply to Vsupply : Saturate  UpperLimit=5  LowerLimit=-5  OutDataTypeStr=single
  "conversion to dutycycle (convert to uint8, overflow will provide reverse polairty magnitued)" : Gain  Gain=255/Vsupply  OutDataTypeStr=uint8
  wires:
  Abs/1 -> "conversion to dutycycle (convert to uint8, overflow will provide reverse polairty magnitued)"/1
  Compare To Zero1/1 -> Digital Output2/1
  Compare To Zero/1 -> Digital Output1/1
  "conversion to dutycycle (convert to uint8, overflow will provide reverse polairty magnitued)"/1 -> PWM/1(In1)
  Saturation -Vsupply to Vsupply/1 -> Abs/1
  Volts/1 -> Saturation -Vsupply to Vsupply/1, Compare To Zero/1, Compare To Zero1/1

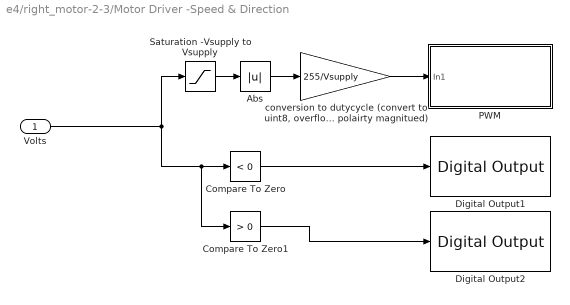
== system e4/right_motor-2-3/Motor Driver -Speed & Direction ==
  Volts : Inport
  Abs : Abs
  Compare To Zero : simulink/Logic and Bit Operations/Compare To Zero  relop=<  OutDataTypeStr=boolean
  Compare To Zero1 : simulink/Logic and Bit Operations/Compare To Zero  relop=>  OutDataTypeStr=boolean
  Digital Output1 : arduinolib/Digital Output  pinNumber=6  blockPlatform=arduino
  Digital Output2 : arduinolib/Digital Output  pinNumber=7  blockPlatform=arduino
  PWM : Subsystem  AncestorBlock=arduinolib/PWM  InitFcn=codertarget.arduinobase.blocks.arduinoBlockInitFcnCallback(gcbh);  mask(Arduino PWM){pinNumber=5, blockPlatform=arduino}
      mask prompts: pinNumber "Pin number:"; blockPlatform "Block platform:"
      mask help:
      | Generate square waveform on the specified analog output pin. The block input controls the duty cycle of the square waveform. An input value of 0 produces a 0 percent duty cycle, and an input value of 255 produces a 100 percent duty cycle. The frequency of the waveform is constant at approximately 490 Hz.
      |
      | Enter the number of the analog output pin. Do not assign the same pin number to multiple blocks within a model.
      mask init:
      | codertarget.arduinobase.blocks.registerPWMBlock(gcbh);
      | codertarget.arduinobase.blocks.arduinoAnalogOutputCallback('MaskInitialization');
      mask Help: eval('codertarget.internal.helpView(''arduinoert'', ''arduinolibarduinopwm'')')
      mask DialogControl Control2 Prompt: View pin map
      mask DialogControl Control2 Callback:
      | file = [codertarget.arduinobase.internal.getBaseSpPkgRootDir filesep 'blocks' filesep 'mex' filesep 'arduinoPinMapping.html'];
      | web(file)
      mask Display:
      | pic=imread('analogoutpwm.png');image(pic,[0.32 0.25 0.35 0.55]);text(0.5, 0.15, 'Pin 5', 'horizontalAlignment', 'center');
      | color('blue');
      | text(0.55, 0.87, 'ARDUINO', 'horizontalAlignment', 'left');
      | color('black');
  Saturation -Vsupply to Vsupply : Saturate  UpperLimit=5  LowerLimit=-5  OutDataTypeStr=single
  "conversion to dutycycle (convert to uint8, overflow will provide reverse polairty magnitued)" : Gain  Gain=255/Vsupply  OutDataTypeStr=uint8
  wires:
  Abs/1 -> "conversion to dutycycle (convert to uint8, overflow will provide reverse polairty magnitued)"/1
  Compare To Zero1/1 -> Digital Output2/1
  Compare To Zero/1 -> Digital Output1/1
  "conversion to dutycycle (convert to uint8, overflow will provide reverse polairty magnitued)"/1 -> PWM/1(In1)
  Saturation -Vsupply to Vsupply/1 -> Abs/1
  Volts/1 -> Saturation -Vsupply to Vsupply/1, Compare To Zero/1, Compare To Zero1/1

== system e4/left_motor-18_19 /Motor Driver -Speed & Direction/PWM ==
  In1 : Inport
  Data Type Conversion : DataTypeConversion  OutDataTypeStr=uint8  SaturateOnIntegerOverflow=on
  PWM : S-Function  FunctionName=arduinoanalogoutput_sfcn  Parameters=pinNumber  SFunctionDeploymentMode=off  EnableBusSupport=off  mask(Arduino Analog Output Core){pinNumber=9}
      mask prompts: pinNumber "Pin number:"
      mask Display: pic=imread('analogoutpwm.png');image(pic,[0.32 0.25 0.35 0.55]);
  wires:
  In1/1 -> Data Type Conversion/1
  Data Type Conversion/1 -> PWM/1

== system e4/right_motor-2-1/Motor Driver -Speed & Direction/PWM ==
  In1 : Inport
  Data Type Conversion : DataTypeConversion  OutDataTypeStr=uint8  SaturateOnIntegerOverflow=on
  PWM : S-Function  FunctionName=arduinoanalogoutput_sfcn  Parameters=pinNumber  SFunctionDeploymentMode=off  EnableBusSupport=off  mask(Arduino Analog Output Core){pinNumber=4}
      mask prompts: pinNumber "Pin number:"
      mask Display: pic=imread('analogoutpwm.png');image(pic,[0.32 0.25 0.35 0.55]);
  wires:
  Data Type Conversion/1 -> PWM/1
  In1/1 -> Data Type Conversion/1

== system e4/right_motor-2-3/Motor Driver -Speed & Direction/PWM ==
  In1 : Inport
  Data Type Conversion : DataTypeConversion  OutDataTypeStr=uint8  SaturateOnIntegerOverflow=on
  PWM : S-Function  FunctionName=arduinoanalogoutput_sfcn  Parameters=pinNumber  SFunctionDeploymentMode=off  EnableBusSupport=off  mask(Arduino Analog Output Core){pinNumber=5}
      mask prompts: pinNumber "Pin number:"
      mask Display: pic=imread('analogoutpwm.png');image(pic,[0.32 0.25 0.35 0.55]);
  wires:
  Data Type Conversion/1 -> PWM/1
  In1/1 -> Data Type Conversion/1
